simulink model "test_latlong_to_xy"  (Simulink 7.6)
settings: Solver=ode45  StartTime=0.0  StopTime=500.0  RelTol=1e-3
libraries: simulink x2
settings Model: Creator=jporter  LastModifiedBy=jporter

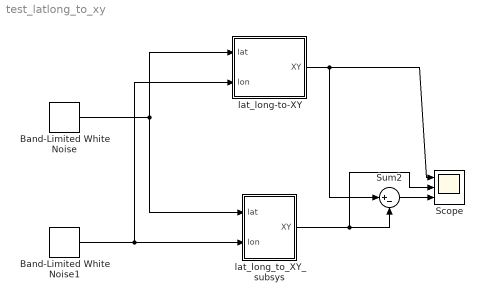
== system test_latlong_to_xy ==
  Band-Limited White Noise : simulink/Sources/Band-Limited White Noise  SystemSampleTime=-1  Cov=[0.1]  Ts=0.01  seed=[23341]
  Band-Limited White Noise1 : simulink/Sources/Band-Limited White Noise  SystemSampleTime=-1  Cov=[0.1]  Ts=0.01  seed=[23341]
  Scope : Scope  NumInputPorts=3
      settings: YMin=-5~-5~-5  YMax=5~5~5
  Sum2 : Sum  Inputs=|+-
  lat_long-to-XY : Stateflow chart  TreatAsAtomicUnit=on
  lat_long_to_XY_subsys : Subsystem
  wires:
  Band-Limited White Noise/1 -> lat_long-to-XY/1(lat), lat_long_to_XY_subsys/1(lat)
  Band-Limited White Noise1/1 -> lat_long-to-XY/2(lon), lat_long_to_XY_subsys/2(lon)
  Sum2/1 -> Scope/3
  lat_long-to-XY/1(XY) -> Scope/1, Sum2/1
  lat_long_to_XY_subsys/1(XY) -> Scope/2, Sum2/2

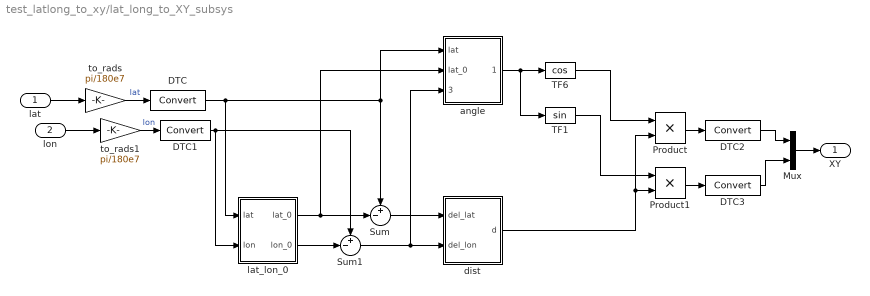
== system test_latlong_to_xy/lat_long_to_XY_subsys ==
  lat : Inport
  lon : Inport  Port=2
  DTC{,1..3} (4 alike) : DataTypeConversion
  Mux : Mux  Inputs=2
  Product : Product  RndMeth=Zero
  Product1 : Product  RndMeth=Zero
  Sum : Sum  Inputs=+-|
  Sum1 : Sum  Inputs=+-|
  TF1 : Trigonometry
  TF6 : Trigonometry  Operator=cos
  angle : Subsystem
  dist : Subsystem
  lat_lon_0 : Subsystem
  to_rads : Gain  Gain=pi/180e7
  to_rads1 : Gain  Gain=pi/180e7
  XY : Outport
  wires:
  to_rads/1 -> DTC/1  "lat"
  to_rads1/1 -> DTC1/1  "lon"
  lat_lon_0/1(lat_0) -> Sum/2, angle/2(lat_0)
  lat_lon_0/2(lon_0) -> Sum1/2
  Sum/1 -> dist/1(del_lat)
  Sum1/1 -> dist/2(del_lon), angle/3(del_lon)
  angle/1(theta) -> TF6/1, TF1/1
  TF6/1 -> Product/1
  TF1/1 -> Product1/1
  dist/1(d) -> Product/2, Product1/2
  Product/1 -> DTC2/1
  Product1/1 -> DTC3/1
  lat/1 -> to_rads/1
  lon/1 -> to_rads1/1
  Mux/1 -> XY/1
  DTC/1 -> lat_lon_0/1(lat), angle/1(lat), Sum/1
  DTC1/1 -> lat_lon_0/2(lon), Sum1/1
  DTC2/1 -> Mux/1
  DTC3/1 -> Mux/2

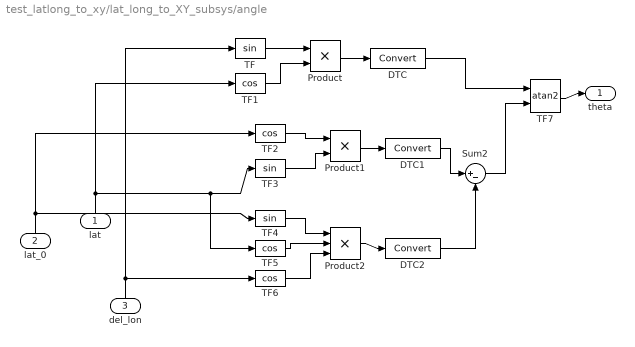
== system test_latlong_to_xy/lat_long_to_XY_subsys/angle ==
  lat : Inport
  lat_0 : Inport  Port=2
  del_lon : Inport  Port=3
  DTC : DataTypeConversion
  DTC1 : DataTypeConversion
  DTC2 : DataTypeConversion
  Product : Product  RndMeth=Zero
  Product1 : Product  RndMeth=Zero
  Product2 : Product  Inputs=3  RndMeth=Zero
  Sum2 : Sum  Inputs=|+-
  TF : Trigonometry
  TF{1..2,5..6} (4 alike) : Trigonometry  Operator=cos
  TF3 : Trigonometry
  TF4 : Trigonometry
  TF7 : Trigonometry  Operator=atan2
  theta : Outport
  wires:
  TF/1 -> Product/1
  TF1/1 -> Product/2
  Product1/1 -> DTC1/1
  Product2/1 -> DTC2/1
  TF2/1 -> Product1/1
  TF3/1 -> Product1/2
  TF4/1 -> Product2/1
  TF5/1 -> Product2/2
  TF6/1 -> Product2/3
  Product/1 -> DTC/1
  Sum2/1 -> TF7/2
  lat/1 -> TF1/1, TF3/1, TF5/1
  lat_0/1 -> TF2/1, TF4/1
  del_lon/1 -> TF/1, TF6/1
  TF7/1 -> theta/1
  DTC/1 -> TF7/1
  DTC1/1 -> Sum2/1
  DTC2/1 -> Sum2/2

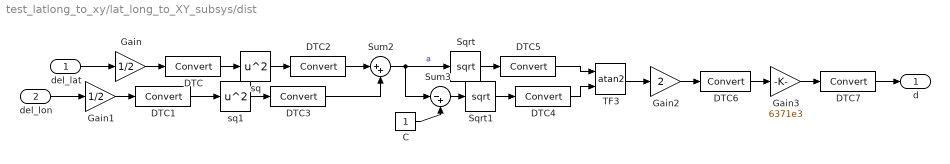
== system test_latlong_to_xy/lat_long_to_XY_subsys/dist ==
  del_lat : Inport
  del_lon : Inport  Port=2
  C : Constant
  DTC{,1..7} (8 alike) : DataTypeConversion
  Gain : Gain  Gain=1/2
  Gain1 : Gain  Gain=1/2
  Gain2 : Gain  Gain=2
  Gain3 : Gain  Gain=6371e3
  Sqrt : Sqrt  SaturateOnIntegerOverflow=on
  Sqrt1 : Sqrt  SaturateOnIntegerOverflow=on
  Sum2 : Sum  Inputs=|++
  Sum3 : Sum  Inputs=|-+
  TF3 : Trigonometry  Operator=atan2
  sq : Math  Operator=square  SaturateOnIntegerOverflow=on
  sq1 : Math  Operator=square  SaturateOnIntegerOverflow=on
  d : Outport
  wires:
  Gain/1 -> DTC/1
  Gain1/1 -> DTC1/1
  sq/1 -> DTC2/1
  sq1/1 -> DTC3/1
  Sum2/1 -> Sum3/1, Sqrt/1  "a"
  C/1 -> Sum3/2
  Sum3/1 -> Sqrt1/1
  Sqrt/1 -> DTC5/1
  Sqrt1/1 -> DTC4/1
  TF3/1 -> Gain2/1
  Gain2/1 -> DTC6/1
  del_lat/1 -> Gain/1
  Gain3/1 -> DTC7/1
  del_lon/1 -> Gain1/1
  DTC/1 -> sq/1
  DTC1/1 -> sq1/1
  DTC2/1 -> Sum2/1
  DTC3/1 -> Sum2/2
  DTC4/1 -> TF3/2
  DTC5/1 -> TF3/1
  DTC6/1 -> Gain3/1
  DTC7/1 -> d/1

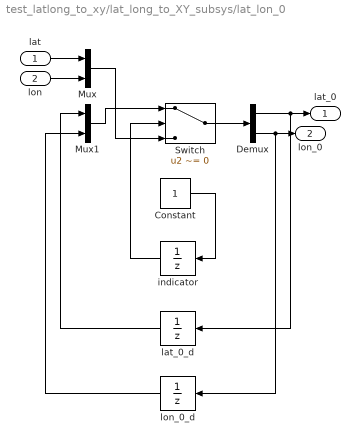
== system test_latlong_to_xy/lat_long_to_XY_subsys/lat_lon_0 ==
  lat : Inport
  lon : Inport  Port=2
  Constant : Constant
  Demux : Demux  Outputs=2
  Mux : Mux  Inputs=2
  Mux1 : Mux  Inputs=2
  Switch : Switch  Criteria=u2 ~= 0
  indicator : UnitDelay  SampleTime=-1
  lat_0_d : UnitDelay  SampleTime=-1
  lon_0_d : UnitDelay  SampleTime=-1
  lat_0 : Outport
  lon_0 : Outport  Port=2
  wires:
  Constant/1 -> indicator/1
  indicator/1 -> Switch/2
  Mux/1 -> Switch/3
  lat_0_d/1 -> Mux1/1
  lon_0_d/1 -> Mux1/2
  Mux1/1 -> Switch/1
  Switch/1 -> Demux/1
  Demux/1 -> lat_0_d/1, lat_0/1
  Demux/2 -> lon_0_d/1, lon_0/1
  lat/1 -> Mux/1
  lon/1 -> Mux/2

== matlab function lat_long-to-XY ==
  data: XY output double size=[2]; lat input double size=[1]; lon input double size=[1]
function XY  = fcn(lat,lon)
%Convert latitude and longitude to relative XY position from an initial
%latitude and longitude reading
    persistent lat_0;
    persistent lon_0;
    R = 6371e3;         %Earth's Radius meters
    lat = lat*pi/180e7; %Convert from 1e-7 degrees to radians
    lon = lon*pi/180e7; %Convert from 1e-7 degrees to radians
    if isempty(lat_0)
        lat_0 = lat;
    end
    if lat_0 == 0
        lat_0 = lat;
    end
    if isempty(lon_0)
        lon_0 = lon;
    end
    if lon_0 == 0
        lon_0 = lon;
    end
    XY = zeros(2,1);
    if (lat_0 ~= 0) && (lon_0 ~= 0)
        %Compute distance between two-points using haversine formula
        del_lat = lat - lat_0;
        del_lon = lon - lon_0;
        a = sin(del_lat/2)^2 + cos(lat)*sin(del_lon/2)^2;
        c = 2*atan2(sqrt(a),sqrt(1-a));
        d = R*c;     %Distance traveled from starting point (0,0) in meters
        yt = sin(del_lon)*cos(lat);
        xt = cos(lat_0)*sin(lat) - sin(lat_0)*cos(lat)*cos(del_lon);
        th = atan2(yt,xt);
        X = d*cos(th);
        Y = d*sin(th);
        XY(1) = X;
        XY(2) = Y;
    end
    
    lat0 = lat_0;
    lon0 = lon_0;
